simulink model "grid_tied_50KW_inverter"  (R2020a)
settings: Solver=VariableStepAuto  StartTime=0.0  StopTime=10.0  RelTol=1e-3
values from neighbouring files (symbols this model uses):
  f = 50    [grid_tie_param.m]
  L = 0.15*Pbase/(2*pi*f)    (= 0.00137891842695)    [grid_tie_param.m]
  RL = (1.5e-3)*Pbase    (= 0.004332)    [grid_tie_param.m]
  Ts_Power = 1/(fs*100)    (= 2.0202020202e-06)    [grid_tie_param.m]
  Vbase = 380    [grid_tie_param.m]
  Vdc = 700    [grid_tie_param.m]
libraries: powerlib x10, powerlib_meascontrol x3
settings Model: Creator=Junaed  LastModifiedBy=Junaed

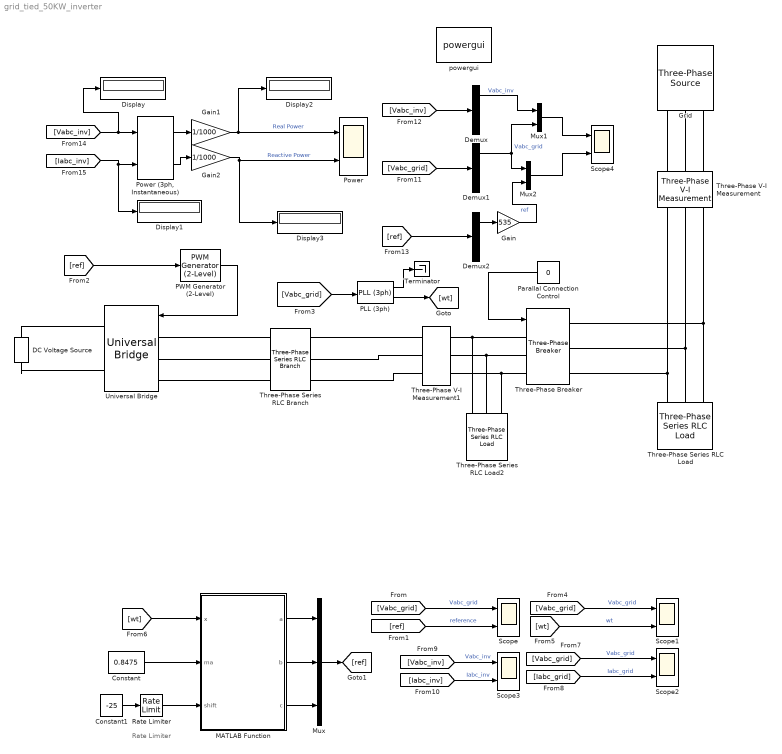
== system grid_tied_50KW_inverter ==
  note: Rate Limiter
  Constant : Constant  Value=0.8475
  Constant1 : Constant  Value=-25
  DC Voltage Source : powerlib/Electrical Sources/DC Voltage Source  Amplitude=Vdc  Measurements=None
  Demux : Demux  Outputs=3
  Demux1 : Demux  Outputs=3
  Demux2 : Demux  Outputs=3
  Display{,1..3} (4 alike) : Display
  Gain : Gain  Gain=535
  Gain1 : Gain  Gain=1/1000
  Gain2 : Gain  Gain=1/1000
  Grid : powerlib/Electrical Sources/Three-Phase Source  InternalConnection=Yg  VoltagePhases=off  Voltage=Vbase  PhaseAngle=0  Voltage_phases=[25e3 25e3 25e3]/sqrt(3)  PhaseAngles_phases=[0 -120 +120]  Frequency=f  NonIdealSource=on  SpecifyImpedance=on  Resistance=0.8929  Inductance=16.58e-3  ShortCircuitLevel=100e6  BaseVoltage=Vbase  XRratio=7  BusType=swing  Pref=10e3  Qref=0  Prefabc=[10e3, 10e3, 10e3]  Qrefabc=[0, 0, 0]  Qmin=-inf  Qmax=inf
  MATLAB Function : MATLAB Function  TreatAsAtomicUnit=on
  Mux : Mux  Inputs=3
  Mux1 : Mux  Inputs=2
  Mux2 : Mux  Inputs=2
  PLL (3ph) : powerlib_meascontrol/PLL/PLL (3ph)  Fmin=45  Par_Init=[0, f]  ParK=[180, 3200, 1]  TcD=1e-4  MaxRateChangeFreq=12  FilterCutOffFreq=25  Ts=Ts_Power  AGC=on
  PWM Generator (2-Level) : powerlib_meascontrol/Pulse & Signal Generators/PWM Generator (2-Level)  ModulatorType=Three-phase bridge (6 pulses)  ModulatorMode=Unsynchronized  Fc=fs  Pc=90  nF=27  MinMax="[ -1  1 ]"  SamplingTechnique=Natural  ModulatingSignals=off  m=0.8  Freq=60  Phase=0  Ts=Ts_Power  ShowCarrierOutport=off
  Parallal Connection Control : Constant  Value=0
  Power : Scope  NumInputPorts=2
  "Power (3ph, Instantaneous)" : powerlib_meascontrol/Measurements/Power (3ph, Instantaneous)
  Rate Limiter : RateLimiter  RisingSlewLimit=100  FallingSlewLimit=-100
  Scope{,1..4} (5 alike) : Scope  NumInputPorts=2
  Terminator : Terminator
  Three-Phase Series RLC Branch : powerlib/Elements/Three-Phase Series RLC Branch  LConnTagsString=A|B|C  RConnTagsString=A|B|C  BranchType=RL  Resistance=RL  Inductance=L  Capacitance=1e-6  Measurements=None
  Three-Phase Series RLC Load : powerlib/Elements/Three-Phase Series RLC Load  LConnTagsString=A|B|C  Configuration=Y (grounded)  NominalVoltage=Vbase  Vabc=[1e3 1e3 1e3]  Vabcp=[1e3 1e3 1e3]  NominalFrequency=f  UnbalancedPower=off  ActivePower=10e3  InductivePower=0  CapacitivePower=0  Pabc=[10e3 9e3 11e3]  QLabc=[100 90 110]  QCabc=[100 90 110]  Pabcp=[10e3 9e3 11e3]  QLabcp=[100 90 110]  QCabcp=[100 90 110]  Measurements=None  LoadType=constant Z
  Three-Phase Series RLC Load2 : powerlib/Elements/Three-Phase Series RLC Load  LConnTagsString=A|B|C  Configuration=Delta  NominalVoltage=Vbase  Vabc=[1e3 1e3 1e3]  Vabcp=[1e3 1e3 1e3]  NominalFrequency=f  UnbalancedPower=off  ActivePower=Pc  InductivePower=0  CapacitivePower=Qc  Pabc=[10e3 9e3 11e3]  QLabc=[100 90 110]  QCabc=[100 90 110]  Pabcp=[10e3 9e3 11e3]  QLabcp=[100 90 110]  QCabcp=[100 90 110]  Measurements=None  LoadType=constant Z
  Three-Phase V-I Measurement : powerlib/Measurements/Three-Phase V-I Measurement  VoltageMeasurement=phase-to-phase  SetLabelV=on  LabelV=Vabc_grid  Vpu=off  VpuLL=off  CurrentMeasurement=yes  SetLabelI=on  LabelI=Iabc_grid  Ipu=off  Pbase=100e6  Vbase=500e3  OutputType=Complex  PhasorSimulation=off  PSBequivalent=0
  Three-Phase V-I Measurement1 : powerlib/Measurements/Three-Phase V-I Measurement  VoltageMeasurement=phase-to-phase  SetLabelV=on  LabelV=Vabc_inv  Vpu=off  VpuLL=off  CurrentMeasurement=yes  SetLabelI=on  LabelI=Iabc_inv  Ipu=off  Pbase=100e6  Vbase=500e3  OutputType=Complex  PhasorSimulation=off  PSBequivalent=0
  Three-Phase Breaker : powerlib/Elements/Three-Phase Breaker  InitialState=open  SwitchA=on  SwitchB=on  SwitchC=on  SwitchTimes="[1/60  5/60]"  External=on  BreakerResistance=0.01  SnubberResistance=1e6  SnubberCapacitance=inf  Measurements=None
  Universal Bridge : powerlib/Power Electronics/Universal Bridge  Arms=3  SnubberResistance=1e6  SnubberCapacitance=inf  Device=IGBT / Diodes  Ron=1e-3  Lon=0  ForwardVoltages="[  0  0  ]"  ForwardVoltage=0  GTOparameters=[ 10e-6 , 20e-6 ]  IGBTparameters=[ 1e-6 , 2e-6 ]  Measurements=None  Measurements_2=None  converterType=Rectifier
  powergui : powerlib/powergui  Priority=1  SimulationMode=Discrete  SampleTime=Ts_Power  frequency=60  Iterations=50  frequencyindice=0  Pbase=100e6  ErrMax=1e-4  UnitsV=kV  UnitsW=MW  buscounter=0  FunctionMessages=off  echomessages=off  EnableUseOfTLC=off  CurrentSourceSwitches=off  DisableSnubberDevices=off  DisableRonSwitches=off  DisableVfSwitches=off  DisplayEquations=off  AutomaticDiscreteSolvers=off  SolverType=Tustin/Backward Euler (TBE)  Interpol=off  ExternalGateDelay=off  methode=off  Ts=100  x0status=blocks  SPID=on  SwTol=0  HookPort=off  NonlinearTolerance=1e-4  nMaxIteration=100  ContinueOnMaxIteration=off  RestoreLinks=warning  ResistiveCurrentMeasurement=off  Frange=[0:2:500]  Ylog=off  Xlog=on  ShowGrid=off  save=off  variable=ZData  structure=0  ZoomFFT=off  StartTime=0.0  cycles=1  DisplayStyle=1  fundamental=60  FreqAxis=off  MaxFrequency=1000  frequencyindicesteady=1  RmsSteady=1  display=off
  wires:
  [Vabc_grid] -> Scope/1  "Vabc_grid"
  [ref] -> Scope/2  "reference"
  PWM Generator (2-Level)/1 -> Universal Bridge/1
  [ref] -> PWM Generator (2-Level)/1
  [Vabc_grid] -> PLL (3ph)/1
  PLL (3ph)/2 -> [wt]
  [wt] -> Scope1/2  "wt"
  [Vabc_grid] -> Scope1/1  "Vabc_grid"
  [wt] -> MATLAB Function/1(x)
  Constant/1 -> MATLAB Function/2(ma)
  Rate Limiter/1 -> MATLAB Function/3(shift)
  Constant1/1 -> Rate Limiter/1
  MATLAB Function/1(a) -> Mux/1
  MATLAB Function/2(b) -> Mux/2
  MATLAB Function/3(c) -> Mux/3
  Mux/1 -> [ref]
  [Iabc_grid] -> Scope2/2  "Iabc_grid"
  [Vabc_grid] -> Scope2/1  "Vabc_grid"
  Parallal Connection Control/1 -> Three-Phase Breaker/1
  [Vabc_inv] -> Scope3/1  "Vabc_inv"
  [Iabc_inv] -> Scope3/2  "Iabc_inv"
  [Vabc_grid] -> Demux1/1
  [Vabc_inv] -> Demux/1
  [ref] -> Demux2/1
  Mux1/1 -> Scope4/1
  Demux/1 -> Mux1/1  "Vabc_inv"
  Demux1/1 -> Mux1/2, Mux2/1  "Vabc_grid"
  Demux2/1 -> Gain/1
  Gain/1 -> Mux2/2  "ref"
  Mux2/1 -> Scope4/2
  [Vabc_inv] -> "Power (3ph, Instantaneous)"/1, Display/1
  "Power (3ph, Instantaneous)"/1 -> Gain1/1
  Gain1/1 -> Display2/1, Power/1  "Real Power"
  Gain2/1 -> Display3/1, Power/2  "Reactive Power"
  PLL (3ph)/1 -> Terminator/1
  [Iabc_inv] -> "Power (3ph, Instantaneous)"/2, Display1/1
  "Power (3ph, Instantaneous)"/2 -> Gain2/1
  connections:
  Three-Phase V-I Measurement/LConn3 -- Grid/RConn3
  Grid/RConn2 -- Three-Phase V-I Measurement/LConn2
  Grid/RConn1 -- Three-Phase V-I Measurement/LConn1
  Three-Phase Series RLC Load/LConn1 -- Three-Phase Breaker/RConn3 -- Three-Phase V-I Measurement/RConn3
  Three-Phase Series RLC Load/LConn2 -- Three-Phase Breaker/RConn2 -- Three-Phase V-I Measurement/RConn2
  Three-Phase V-I Measurement/RConn1 -- Three-Phase Series RLC Load/LConn3 -- Three-Phase Breaker/RConn1
  DC Voltage Source/LConn1 -- Universal Bridge/RConn2
  DC Voltage Source/RConn1 -- Universal Bridge/RConn1
  Three-Phase Series RLC Branch/LConn1 -- Universal Bridge/LConn1
  Three-Phase Series RLC Branch/LConn2 -- Universal Bridge/LConn2
  Universal Bridge/LConn3 -- Three-Phase Series RLC Branch/LConn3
  Three-Phase V-I Measurement1/LConn1 -- Three-Phase Series RLC Branch/RConn1
  Three-Phase V-I Measurement1/LConn2 -- Three-Phase Series RLC Branch/RConn2
  Three-Phase V-I Measurement1/LConn3 -- Three-Phase Series RLC Branch/RConn3
  Three-Phase Breaker/LConn1 -- Three-Phase Series RLC Load2/LConn1 -- Three-Phase V-I Measurement1/RConn1
  Three-Phase Breaker/LConn2 -- Three-Phase Series RLC Load2/LConn2 -- Three-Phase V-I Measurement1/RConn2
  Three-Phase Breaker/LConn3 -- Three-Phase Series RLC Load2/LConn3 -- Three-Phase V-I Measurement1/RConn3

== matlab function grid_tied_50KW_inverter/MATLAB Function ==
  data: x input; a output; ma input; shift input; b output; c output
function [a,b,c] = ref_generator(x,ma,shift)
%x=wt
shift_k =shift*pi/180 ;         %degree to rad/s
a=(ma*(sin((x)+shift_k)));      %phase A refernce voltage equation
b=(ma*(sin((x)+shift_k-(2*pi/3))));
c=(ma*(sin((x)+shift_k+(2*pi/3))));
end
